simulink model "dsaviorsim"  (R2018a)
settings: Solver=ode45  StartTime=0.0  StopTime=100  RelTol=1e-3  EnableMultiTasking=on
settings Model: Creator=SAITFASKA  LastModifiedBy=admin
settings DataIOCC: LimitDataPoints=on  SaveFormat=Array
settings OptimizationCC: LifeSpan=inf
settings DebuggingCC: UnderspecifiedInitializationDetection=Classic  MergeDetectMultiDrivingBlocksExec=none  SolverPrmCheckMsg=warning  StateNameClashWarn=warning  SFUnexpectedBacktrackingDiag=warning  SFNoUnconditionalDefaultTransitionDiag=warning  SFExecutionAtInitializationDiag=none
settings HardwareCC: ProdBitPerPointer=32  ProdBitPerSizeT=32  ProdBitPerPtrDiffT=32  ProdLargestAtomicFloat=None  ProdIntDivRoundTo=Undefined  ProdEndianess=Unspecified  ProdWordSize=32  ProdHWDeviceType=32-bit Generic
settings ModelReferenceCC: PropagateSignalLabelsOutOfModel=off
settings CodeAppCC: StateflowObjectComments=on
settings GRTTargetCC: TargetLangStandard=C89/C90 (ANSI)  GeneratePreprocessorConditionals=Disable all
settings ConfigComp: CovMetricSettings=dw  CovHtmlReporting=on  CovSaveCumulativeToWorkspaceVar=on  CovSaveSingleToWorkspaceVar=on  CovExternalEMLEnable=off

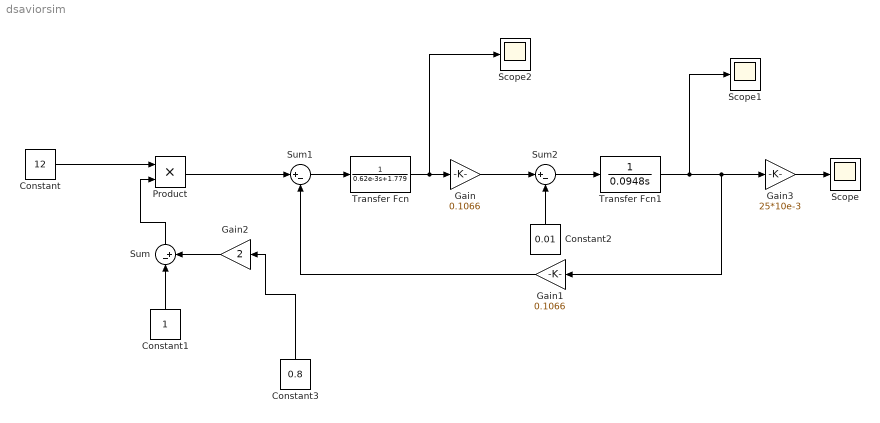
== system dsaviorsim ==
  Constant : Constant  Value=12
  Constant1 : Constant
  Constant2 : Constant  Value=0.01
  Constant3 : Constant  Value=0.8
  Gain : Gain  Gain=0.1066
  Gain1 : Gain  Gain=0.1066
  Gain2 : Gain  Gain=2
  Gain3 : Gain  Gain=25*10e-3
  Product : Product
  Scope : Scope
  Scope1 : Scope
  Scope2 : Scope
  Sum : Sum  Inputs=|-+
  Sum1 : Sum  Inputs=|+-
  Sum2 : Sum  Inputs=|+-
  Transfer Fcn : TransferFcn  Denominator="[0.62e-3  1.779]"
  Transfer Fcn1 : TransferFcn  Denominator=[ 0.0948 0]
  wires:
  Constant1/1 -> Sum/1
  Gain2/1 -> Sum/2
  Sum/1 -> Product/2
  Product/1 -> Sum1/1
  Sum1/1 -> Transfer Fcn/1
  Transfer Fcn/1 -> Scope2/1, Gain/1
  Gain/1 -> Sum2/1
  Constant2/1 -> Sum2/2
  Gain1/1 -> Sum1/2
  Gain3/1 -> Scope/1
  Constant3/1 -> Gain2/1
  Sum2/1 -> Transfer Fcn1/1
  Transfer Fcn1/1 -> Scope1/1, Gain1/1, Gain3/1
  Constant/1 -> Product/1
